simulink model "Q2_Part4"  (R2020a)
settings: Solver=VariableStepAuto  StartTime=0.0  StopTime=10.0  RelTol=1e-3
settings Model: Creator=golnazsalehi  LastModifiedBy=golnazsalehi

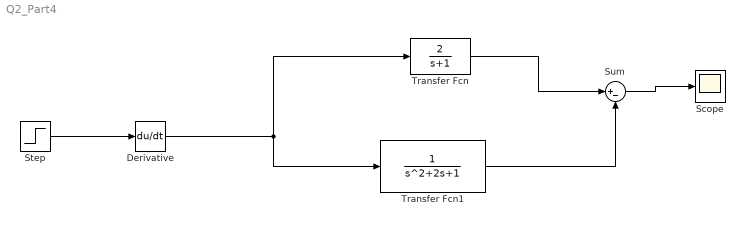
== system Q2_Part4 ==
  Derivative : Derivative
  Scope : Scope
  Step : Step  Time=0.001  SampleTime=0
  Sum : Sum  Inputs=|+-
  Transfer Fcn : TransferFcn  Numerator=[2]  Denominator=[1 1]
  Transfer Fcn1 : TransferFcn  Denominator=[1 2 1]
  wires:
  Step/1 -> Derivative/1
  Transfer Fcn1/1 -> Sum/2
  Transfer Fcn/1 -> Sum/1
  Derivative/1 -> Transfer Fcn1/1, Transfer Fcn/1
  Sum/1 -> Scope/1
